simulink model "RobotX_SLAMonly"  (R2014a)
settings: Solver=FixedStepDiscrete  StartTime=0.0  StopTime=inf  FixedStep=.25  RelTol=1e-3
undefined symbols (not defined in the file): Com1, Com2, Com3, Com4, DiscIntNeverNeededParam, standard
libraries: xpcseriallib x11, simulink x3, slrtlib x3, dspmtrx3 x2, speedgoatlib x1, speedgoatlib_IO102 x1
(part 9 of 15)

== system RobotX_SLAMonly/Main FSM/SLAM/Models for prediction/Model40 ==
  X : Inport
  Y : Inport  Port=2
  Psi : Inport  Port=3
  Nav Messages : Inport  Port=4
  Bus Selector : BusSelector  OutputSignals=Velocity.u,Velocity.v,Velocity.r,Port.PtThrust,Port.PtAzimuth,Stbd.StThrust,Stbd.StAzimuth
  Data Store Read : DataStoreRead  DataStoreName=noiseLevel
  Demux : Demux  Outputs=3
  Discrete-Time Integrator1 : DiscreteIntegrator  SampleTime=-1  ICPrevOutput=DiscIntNeverNeededParam  ICPrevScaledInput=DiscIntNeverNeededParam
  Dynamic Model : MATLAB Function  TreatAsAtomicUnit=on
  Mux : Mux  Inputs=3
  Mux1 : Mux  Inputs=3
  Non-Holonomic Constraint : MATLAB Function  TreatAsAtomicUnit=on
  Port Thruster Model : MATLAB Function  TreatAsAtomicUnit=on
  Stbd Thruster Model : MATLAB Function  TreatAsAtomicUnit=on
  Sum : Sum  Inputs=|++|
  enabled : Constant
  move_part : MATLAB Function  TreatAsAtomicUnit=on
  NEyaw : Outport
  wires:
  Sum/1 -> Demux/1  "Forces"
  Bus Selector/2 -> Non-Holonomic Constraint/6(v), Dynamic Model/5(v)  "<v>"
  Bus Selector/1 -> Non-Holonomic Constraint/5(u), Dynamic Model/4(u)  "<u>"
  Psi/1 -> Non-Holonomic Constraint/8(psi), Dynamic Model/6(psi)
  Demux/2 -> Dynamic Model/2(F_sway)
  Demux/3 -> Dynamic Model/3(Torque)
  Demux/1 -> Dynamic Model/1(F_surge)
  Mux/1 -> Sum/2
  Stbd Thruster Model/1(F_surge) -> Mux/1
  Stbd Thruster Model/3(Torque) -> Mux/3
  Stbd Thruster Model/2(F_sway) -> Mux/2
  Mux1/1 -> Sum/1
  Port Thruster Model/2(F_sway) -> Mux1/2
  Port Thruster Model/1(F_surge) -> Mux1/1
  Port Thruster Model/3(Torque) -> Mux1/3
  Dynamic Model/1(surgeAccel) -> Non-Holonomic Constraint/2(surgeAccel)
  Dynamic Model/2(swayAccel) -> Non-Holonomic Constraint/3(swayAccel)
  Dynamic Model/3(yawAccel) -> Non-Holonomic Constraint/4(YawAccel)
  Y/1 -> Non-Holonomic Constraint/10(Y)
  X/1 -> Non-Holonomic Constraint/9(X)
  Bus Selector/3 -> Non-Holonomic Constraint/7(gyrz)  "<r>"
  Non-Holonomic Constraint/1(NEyaw) -> NEyaw/1
  enabled/1 -> Discrete-Time Integrator1/1
  Discrete-Time Integrator1/1 -> Non-Holonomic Constraint/1(time)
  Nav Messages/1 -> Bus Selector/1
  Bus Selector/4 -> move_part/1(PtThrust)  "<PtThrust>"
  Bus Selector/5 -> move_part/2(PtAzimuth)  "<PtAzimuth>"
  Bus Selector/7 -> move_part/4(StAzimuth)  "<StAzimuth>"
  Bus Selector/6 -> move_part/3(StThrust)  "<StThrust>"
  move_part/1(portMP) -> Port Thruster Model/1(portMP)
  move_part/2(portAzimuth) -> Port Thruster Model/2(portAzimuth)
  move_part/3(stbdMP) -> Stbd Thruster Model/1(stbdMP)
  move_part/4(stbdAzimuth) -> Stbd Thruster Model/2(stbdAzimuth)
  Data Store Read/1 -> move_part/5(noiseLevel)

== system RobotX_SLAMonly/Main FSM/SLAM/Models for prediction/Model41 ==
  X : Inport
  Y : Inport  Port=2
  Psi : Inport  Port=3
  Nav Messages : Inport  Port=4
  Bus Selector : BusSelector  OutputSignals=Velocity.u,Velocity.v,Velocity.r,Port.PtThrust,Port.PtAzimuth,Stbd.StThrust,Stbd.StAzimuth
  Data Store Read : DataStoreRead  DataStoreName=noiseLevel
  Demux : Demux  Outputs=3
  Discrete-Time Integrator1 : DiscreteIntegrator  SampleTime=-1  ICPrevOutput=DiscIntNeverNeededParam  ICPrevScaledInput=DiscIntNeverNeededParam
  Dynamic Model : MATLAB Function  TreatAsAtomicUnit=on
  Mux : Mux  Inputs=3
  Mux1 : Mux  Inputs=3
  Non-Holonomic Constraint : MATLAB Function  TreatAsAtomicUnit=on
  Port Thruster Model : MATLAB Function  TreatAsAtomicUnit=on
  Stbd Thruster Model : MATLAB Function  TreatAsAtomicUnit=on
  Sum : Sum  Inputs=|++|
  enabled : Constant
  move_part : MATLAB Function  TreatAsAtomicUnit=on
  NEyaw : Outport
  wires:
  Sum/1 -> Demux/1  "Forces"
  Bus Selector/2 -> Non-Holonomic Constraint/6(v), Dynamic Model/5(v)  "<v>"
  Bus Selector/1 -> Non-Holonomic Constraint/5(u), Dynamic Model/4(u)  "<u>"
  Psi/1 -> Non-Holonomic Constraint/8(psi), Dynamic Model/6(psi)
  Demux/2 -> Dynamic Model/2(F_sway)
  Demux/3 -> Dynamic Model/3(Torque)
  Demux/1 -> Dynamic Model/1(F_surge)
  Mux/1 -> Sum/2
  Stbd Thruster Model/1(F_surge) -> Mux/1
  Stbd Thruster Model/3(Torque) -> Mux/3
  Stbd Thruster Model/2(F_sway) -> Mux/2
  Mux1/1 -> Sum/1
  Port Thruster Model/2(F_sway) -> Mux1/2
  Port Thruster Model/1(F_surge) -> Mux1/1
  Port Thruster Model/3(Torque) -> Mux1/3
  Dynamic Model/1(surgeAccel) -> Non-Holonomic Constraint/2(surgeAccel)
  Dynamic Model/2(swayAccel) -> Non-Holonomic Constraint/3(swayAccel)
  Dynamic Model/3(yawAccel) -> Non-Holonomic Constraint/4(YawAccel)
  Y/1 -> Non-Holonomic Constraint/10(Y)
  X/1 -> Non-Holonomic Constraint/9(X)
  Bus Selector/3 -> Non-Holonomic Constraint/7(gyrz)  "<r>"
  Non-Holonomic Constraint/1(NEyaw) -> NEyaw/1
  enabled/1 -> Discrete-Time Integrator1/1
  Discrete-Time Integrator1/1 -> Non-Holonomic Constraint/1(time)
  Nav Messages/1 -> Bus Selector/1
  Bus Selector/4 -> move_part/1(PtThrust)  "<PtThrust>"
  Bus Selector/5 -> move_part/2(PtAzimuth)  "<PtAzimuth>"
  Bus Selector/7 -> move_part/4(StAzimuth)  "<StAzimuth>"
  Bus Selector/6 -> move_part/3(StThrust)  "<StThrust>"
  move_part/1(portMP) -> Port Thruster Model/1(portMP)
  move_part/2(portAzimuth) -> Port Thruster Model/2(portAzimuth)
  move_part/3(stbdMP) -> Stbd Thruster Model/1(stbdMP)
  move_part/4(stbdAzimuth) -> Stbd Thruster Model/2(stbdAzimuth)
  Data Store Read/1 -> move_part/5(noiseLevel)

== system RobotX_SLAMonly/Main FSM/SLAM/Models for prediction/Model42 ==
  X : Inport
  Y : Inport  Port=2
  Psi : Inport  Port=3
  Nav Messages : Inport  Port=4
  Bus Selector : BusSelector  OutputSignals=Velocity.u,Velocity.v,Velocity.r,Port.PtThrust,Port.PtAzimuth,Stbd.StThrust,Stbd.StAzimuth
  Data Store Read : DataStoreRead  DataStoreName=noiseLevel
  Demux : Demux  Outputs=3
  Discrete-Time Integrator1 : DiscreteIntegrator  SampleTime=-1  ICPrevOutput=DiscIntNeverNeededParam  ICPrevScaledInput=DiscIntNeverNeededParam
  Dynamic Model : MATLAB Function  TreatAsAtomicUnit=on
  Mux : Mux  Inputs=3
  Mux1 : Mux  Inputs=3
  Non-Holonomic Constraint : MATLAB Function  TreatAsAtomicUnit=on
  Port Thruster Model : MATLAB Function  TreatAsAtomicUnit=on
  Stbd Thruster Model : MATLAB Function  TreatAsAtomicUnit=on
  Sum : Sum  Inputs=|++|
  enabled : Constant
  move_part : MATLAB Function  TreatAsAtomicUnit=on
  NEyaw : Outport
  wires:
  Sum/1 -> Demux/1  "Forces"
  Bus Selector/2 -> Non-Holonomic Constraint/6(v), Dynamic Model/5(v)  "<v>"
  Bus Selector/1 -> Non-Holonomic Constraint/5(u), Dynamic Model/4(u)  "<u>"
  Psi/1 -> Non-Holonomic Constraint/8(psi), Dynamic Model/6(psi)
  Demux/2 -> Dynamic Model/2(F_sway)
  Demux/3 -> Dynamic Model/3(Torque)
  Demux/1 -> Dynamic Model/1(F_surge)
  Mux/1 -> Sum/2
  Stbd Thruster Model/1(F_surge) -> Mux/1
  Stbd Thruster Model/3(Torque) -> Mux/3
  Stbd Thruster Model/2(F_sway) -> Mux/2
  Mux1/1 -> Sum/1
  Port Thruster Model/2(F_sway) -> Mux1/2
  Port Thruster Model/1(F_surge) -> Mux1/1
  Port Thruster Model/3(Torque) -> Mux1/3
  Dynamic Model/1(surgeAccel) -> Non-Holonomic Constraint/2(surgeAccel)
  Dynamic Model/2(swayAccel) -> Non-Holonomic Constraint/3(swayAccel)
  Dynamic Model/3(yawAccel) -> Non-Holonomic Constraint/4(YawAccel)
  Y/1 -> Non-Holonomic Constraint/10(Y)
  X/1 -> Non-Holonomic Constraint/9(X)
  Bus Selector/3 -> Non-Holonomic Constraint/7(gyrz)  "<r>"
  Non-Holonomic Constraint/1(NEyaw) -> NEyaw/1
  enabled/1 -> Discrete-Time Integrator1/1
  Discrete-Time Integrator1/1 -> Non-Holonomic Constraint/1(time)
  Nav Messages/1 -> Bus Selector/1
  Bus Selector/4 -> move_part/1(PtThrust)  "<PtThrust>"
  Bus Selector/5 -> move_part/2(PtAzimuth)  "<PtAzimuth>"
  Bus Selector/7 -> move_part/4(StAzimuth)  "<StAzimuth>"
  Bus Selector/6 -> move_part/3(StThrust)  "<StThrust>"
  move_part/1(portMP) -> Port Thruster Model/1(portMP)
  move_part/2(portAzimuth) -> Port Thruster Model/2(portAzimuth)
  move_part/3(stbdMP) -> Stbd Thruster Model/1(stbdMP)
  move_part/4(stbdAzimuth) -> Stbd Thruster Model/2(stbdAzimuth)
  Data Store Read/1 -> move_part/5(noiseLevel)

== system RobotX_SLAMonly/Main FSM/SLAM/Models for prediction/Model43 ==
  X : Inport
  Y : Inport  Port=2
  Psi : Inport  Port=3
  Nav Messages : Inport  Port=4
  Bus Selector : BusSelector  OutputSignals=Velocity.u,Velocity.v,Velocity.r,Port.PtThrust,Port.PtAzimuth,Stbd.StThrust,Stbd.StAzimuth
  Data Store Read : DataStoreRead  DataStoreName=noiseLevel
  Demux : Demux  Outputs=3
  Discrete-Time Integrator1 : DiscreteIntegrator  SampleTime=-1  ICPrevOutput=DiscIntNeverNeededParam  ICPrevScaledInput=DiscIntNeverNeededParam
  Dynamic Model : MATLAB Function  TreatAsAtomicUnit=on
  Mux : Mux  Inputs=3
  Mux1 : Mux  Inputs=3
  Non-Holonomic Constraint : MATLAB Function  TreatAsAtomicUnit=on
  Port Thruster Model : MATLAB Function  TreatAsAtomicUnit=on
  Stbd Thruster Model : MATLAB Function  TreatAsAtomicUnit=on
  Sum : Sum  Inputs=|++|
  enabled : Constant
  move_part : MATLAB Function  TreatAsAtomicUnit=on
  NEyaw : Outport
  wires:
  Sum/1 -> Demux/1  "Forces"
  Bus Selector/2 -> Non-Holonomic Constraint/6(v), Dynamic Model/5(v)  "<v>"
  Bus Selector/1 -> Non-Holonomic Constraint/5(u), Dynamic Model/4(u)  "<u>"
  Psi/1 -> Non-Holonomic Constraint/8(psi), Dynamic Model/6(psi)
  Demux/2 -> Dynamic Model/2(F_sway)
  Demux/3 -> Dynamic Model/3(Torque)
  Demux/1 -> Dynamic Model/1(F_surge)
  Mux/1 -> Sum/2
  Stbd Thruster Model/1(F_surge) -> Mux/1
  Stbd Thruster Model/3(Torque) -> Mux/3
  Stbd Thruster Model/2(F_sway) -> Mux/2
  Mux1/1 -> Sum/1
  Port Thruster Model/2(F_sway) -> Mux1/2
  Port Thruster Model/1(F_surge) -> Mux1/1
  Port Thruster Model/3(Torque) -> Mux1/3
  Dynamic Model/1(surgeAccel) -> Non-Holonomic Constraint/2(surgeAccel)
  Dynamic Model/2(swayAccel) -> Non-Holonomic Constraint/3(swayAccel)
  Dynamic Model/3(yawAccel) -> Non-Holonomic Constraint/4(YawAccel)
  Y/1 -> Non-Holonomic Constraint/10(Y)
  X/1 -> Non-Holonomic Constraint/9(X)
  Bus Selector/3 -> Non-Holonomic Constraint/7(gyrz)  "<r>"
  Non-Holonomic Constraint/1(NEyaw) -> NEyaw/1
  enabled/1 -> Discrete-Time Integrator1/1
  Discrete-Time Integrator1/1 -> Non-Holonomic Constraint/1(time)
  Nav Messages/1 -> Bus Selector/1
  Bus Selector/4 -> move_part/1(PtThrust)  "<PtThrust>"
  Bus Selector/5 -> move_part/2(PtAzimuth)  "<PtAzimuth>"
  Bus Selector/7 -> move_part/4(StAzimuth)  "<StAzimuth>"
  Bus Selector/6 -> move_part/3(StThrust)  "<StThrust>"
  move_part/1(portMP) -> Port Thruster Model/1(portMP)
  move_part/2(portAzimuth) -> Port Thruster Model/2(portAzimuth)
  move_part/3(stbdMP) -> Stbd Thruster Model/1(stbdMP)
  move_part/4(stbdAzimuth) -> Stbd Thruster Model/2(stbdAzimuth)
  Data Store Read/1 -> move_part/5(noiseLevel)

== system RobotX_SLAMonly/Main FSM/SLAM/Models for prediction/Model44 ==
  X : Inport
  Y : Inport  Port=2
  Psi : Inport  Port=3
  Nav Messages : Inport  Port=4
  Bus Selector : BusSelector  OutputSignals=Velocity.u,Velocity.v,Velocity.r,Port.PtThrust,Port.PtAzimuth,Stbd.StThrust,Stbd.StAzimuth
  Data Store Read : DataStoreRead  DataStoreName=noiseLevel
  Demux : Demux  Outputs=3
  Discrete-Time Integrator1 : DiscreteIntegrator  SampleTime=-1  ICPrevOutput=DiscIntNeverNeededParam  ICPrevScaledInput=DiscIntNeverNeededParam
  Dynamic Model : MATLAB Function  TreatAsAtomicUnit=on
  Mux : Mux  Inputs=3
  Mux1 : Mux  Inputs=3
  Non-Holonomic Constraint : MATLAB Function  TreatAsAtomicUnit=on
  Port Thruster Model : MATLAB Function  TreatAsAtomicUnit=on
  Stbd Thruster Model : MATLAB Function  TreatAsAtomicUnit=on
  Sum : Sum  Inputs=|++|
  enabled : Constant
  move_part : MATLAB Function  TreatAsAtomicUnit=on
  NEyaw : Outport
  wires:
  Sum/1 -> Demux/1  "Forces"
  Bus Selector/2 -> Non-Holonomic Constraint/6(v), Dynamic Model/5(v)  "<v>"
  Bus Selector/1 -> Non-Holonomic Constraint/5(u), Dynamic Model/4(u)  "<u>"
  Psi/1 -> Non-Holonomic Constraint/8(psi), Dynamic Model/6(psi)
  Demux/2 -> Dynamic Model/2(F_sway)
  Demux/3 -> Dynamic Model/3(Torque)
  Demux/1 -> Dynamic Model/1(F_surge)
  Mux/1 -> Sum/2
  Stbd Thruster Model/1(F_surge) -> Mux/1
  Stbd Thruster Model/3(Torque) -> Mux/3
  Stbd Thruster Model/2(F_sway) -> Mux/2
  Mux1/1 -> Sum/1
  Port Thruster Model/2(F_sway) -> Mux1/2
  Port Thruster Model/1(F_surge) -> Mux1/1
  Port Thruster Model/3(Torque) -> Mux1/3
  Dynamic Model/1(surgeAccel) -> Non-Holonomic Constraint/2(surgeAccel)
  Dynamic Model/2(swayAccel) -> Non-Holonomic Constraint/3(swayAccel)
  Dynamic Model/3(yawAccel) -> Non-Holonomic Constraint/4(YawAccel)
  Y/1 -> Non-Holonomic Constraint/10(Y)
  X/1 -> Non-Holonomic Constraint/9(X)
  Bus Selector/3 -> Non-Holonomic Constraint/7(gyrz)  "<r>"
  Non-Holonomic Constraint/1(NEyaw) -> NEyaw/1
  enabled/1 -> Discrete-Time Integrator1/1
  Discrete-Time Integrator1/1 -> Non-Holonomic Constraint/1(time)
  Nav Messages/1 -> Bus Selector/1
  Bus Selector/4 -> move_part/1(PtThrust)  "<PtThrust>"
  Bus Selector/5 -> move_part/2(PtAzimuth)  "<PtAzimuth>"
  Bus Selector/7 -> move_part/4(StAzimuth)  "<StAzimuth>"
  Bus Selector/6 -> move_part/3(StThrust)  "<StThrust>"
  move_part/1(portMP) -> Port Thruster Model/1(portMP)
  move_part/2(portAzimuth) -> Port Thruster Model/2(portAzimuth)
  move_part/3(stbdMP) -> Stbd Thruster Model/1(stbdMP)
  move_part/4(stbdAzimuth) -> Stbd Thruster Model/2(stbdAzimuth)
  Data Store Read/1 -> move_part/5(noiseLevel)

== system RobotX_SLAMonly/Main FSM/SLAM/Models for prediction/Model45 ==
  X : Inport
  Y : Inport  Port=2
  Psi : Inport  Port=3
  Nav Messages : Inport  Port=4
  Bus Selector : BusSelector  OutputSignals=Velocity.u,Velocity.v,Velocity.r,Port.PtThrust,Port.PtAzimuth,Stbd.StThrust,Stbd.StAzimuth
  Data Store Read : DataStoreRead  DataStoreName=noiseLevel
  Demux : Demux  Outputs=3
  Discrete-Time Integrator1 : DiscreteIntegrator  SampleTime=-1  ICPrevOutput=DiscIntNeverNeededParam  ICPrevScaledInput=DiscIntNeverNeededParam
  Dynamic Model : MATLAB Function  TreatAsAtomicUnit=on
  Mux : Mux  Inputs=3
  Mux1 : Mux  Inputs=3
  Non-Holonomic Constraint : MATLAB Function  TreatAsAtomicUnit=on
  Port Thruster Model : MATLAB Function  TreatAsAtomicUnit=on
  Stbd Thruster Model : MATLAB Function  TreatAsAtomicUnit=on
  Sum : Sum  Inputs=|++|
  enabled : Constant
  move_part : MATLAB Function  TreatAsAtomicUnit=on
  NEyaw : Outport
  wires:
  Sum/1 -> Demux/1  "Forces"
  Bus Selector/2 -> Non-Holonomic Constraint/6(v), Dynamic Model/5(v)  "<v>"
  Bus Selector/1 -> Non-Holonomic Constraint/5(u), Dynamic Model/4(u)  "<u>"
  Psi/1 -> Non-Holonomic Constraint/8(psi), Dynamic Model/6(psi)
  Demux/2 -> Dynamic Model/2(F_sway)
  Demux/3 -> Dynamic Model/3(Torque)
  Demux/1 -> Dynamic Model/1(F_surge)
  Mux/1 -> Sum/2
  Stbd Thruster Model/1(F_surge) -> Mux/1
  Stbd Thruster Model/3(Torque) -> Mux/3
  Stbd Thruster Model/2(F_sway) -> Mux/2
  Mux1/1 -> Sum/1
  Port Thruster Model/2(F_sway) -> Mux1/2
  Port Thruster Model/1(F_surge) -> Mux1/1
  Port Thruster Model/3(Torque) -> Mux1/3
  Dynamic Model/1(surgeAccel) -> Non-Holonomic Constraint/2(surgeAccel)
  Dynamic Model/2(swayAccel) -> Non-Holonomic Constraint/3(swayAccel)
  Dynamic Model/3(yawAccel) -> Non-Holonomic Constraint/4(YawAccel)
  Y/1 -> Non-Holonomic Constraint/10(Y)
  X/1 -> Non-Holonomic Constraint/9(X)
  Bus Selector/3 -> Non-Holonomic Constraint/7(gyrz)  "<r>"
  Non-Holonomic Constraint/1(NEyaw) -> NEyaw/1
  enabled/1 -> Discrete-Time Integrator1/1
  Discrete-Time Integrator1/1 -> Non-Holonomic Constraint/1(time)
  Nav Messages/1 -> Bus Selector/1
  Bus Selector/4 -> move_part/1(PtThrust)  "<PtThrust>"
  Bus Selector/5 -> move_part/2(PtAzimuth)  "<PtAzimuth>"
  Bus Selector/7 -> move_part/4(StAzimuth)  "<StAzimuth>"
  Bus Selector/6 -> move_part/3(StThrust)  "<StThrust>"
  move_part/1(portMP) -> Port Thruster Model/1(portMP)
  move_part/2(portAzimuth) -> Port Thruster Model/2(portAzimuth)
  move_part/3(stbdMP) -> Stbd Thruster Model/1(stbdMP)
  move_part/4(stbdAzimuth) -> Stbd Thruster Model/2(stbdAzimuth)
  Data Store Read/1 -> move_part/5(noiseLevel)

== matlab function RobotX_SLAMonly/Main FSM/Path/A Star (Held Length) ==
  data: relPose input; Path output; obGrid input; targetPt input
function Path  = AStarHeldLengthDebug( relPose, obGrid, targetPt )
%Written By Anderson Lebbad on August 27, 2014
%Last Edited on:

%This funtion executes an A* method for path planning given the current
%position of the vessel, the target position for the vessel to reach, and
%a map of obstacles to avoid. The A* method is well documented here:
% www.policyalmanac.org/games/aStarTutorial.htm

%% Define list sizes
[m,n] = size(obGrid);
gridPts = m*n;

%Initialize a path output variable
Path = nan(gridPts,2);
%Initialize variable to track if a solution has been found
solution_found = 0;

%Track the XY coordinates of each point to be evaluated
open_list_XY = nan(gridPts,2);
%Track the calculated F, G, and H weights (where G is the movement cost to
%get to the point, H is the Hypothetical cost to reach the target from that
%point before the full path is evaluated, and F is the sum of both G and H
%costs) for the points being evaluated
open_list_FGH = nan(gridPts,3);
%Track the coordinates of the parent for each of the points being evaluated
open_list_parent = nan(gridPts,2);

%Track the XY coordinates of each point that has been fully evaluated
closed_list_XY = nan(gridPts,2);
%Track the parent coordinate of each point that has been fully evaluated
closed_list_parent = nan(gridPts,2);
emptyClosed = find(isnan(closed_list_XY(:,1)));

%Relative indices to neighboring points of the square, to be used for
%evaluating potential candidates for the open list
neighbors_XY = [-1,-1;-1,0;-1,1;0,1;1,1;1,0;1,-1;0,-1];
neighbors_G = [14;10;14;10;14;10;14;10];

%Make the current pose (in the relative coordinates of the field) the first
%point in the open list
open_list_XY(1,:) = relPose;
current_XY = relPose;
%Set movement cost of this point to zero
open_list_FGH(1,2) = 0;
%Calculate hypothetical cost
open_list_FGH(1,3) = 10*(abs(targetPt(1)-relPose(1))+abs(targetPt(2)-relPose(2)));
%Sum is full cost
open_list_FGH(1,1) = open_list_FGH(1,2) + open_list_FGH(1,3);

%Create a list of invalid pts
%obstacles are invalid
[row, col] = find(obGrid == -1);
%outside the edges are invalid
left = [0:m+1;zeros(1,m+2)]';
right = [0:m+1;(n+1)*ones(1,m+2)]';
bottom = [zeros(1,n);1:n]';
top = [(m+1)*ones(1,n);1:n]';
invalid_pts = [row,col;left;right;bottom;top];
invalid_pts = sortrows(invalid_pts);
%Loop while there are points on the open list
while sum(~isnan(open_list_XY(:,1))) >= 1
    %% Current Square
    
    %Find the lowest F cost square on the open list, checking newer entries
    %over older. This is done by flipping the list up/down to get newer
    %entries to evaluate first. This is marked as the current square
    [~,idxI] = min(flipud(open_list_FGH(:,1)));
    CurrentSquare = gridPts - idxI(1) + 1;
    current_XY = open_list_XY(CurrentSquare,:);
    current_G = open_list_FGH(CurrentSquare,2);
    
    %Find the first empty element in the closed list, and replace the place
    %holder with the information for the current square
    emptyClosed = find(isnan(closed_list_XY(:,1)));
    closed_list_XY(emptyClosed(1),:) = current_XY;
    closed_list_parent(emptyClosed(1),:) = open_list_parent(CurrentSquare,:);
    %Remove the current square from the open list now that it is on the
    %closed list
    open_list_XY(CurrentSquare,:) = NaN;
    open_list_FGH(CurrentSquare,:) = NaN;
    open_list_parent(CurrentSquare,:) = NaN;
    
    %If the current point that just got added to the closed list is the
    %target point, exit the loop because a complete path can be traced
    if (current_XY(1) == targetPt(1)) && (current_XY(2) == targetPt(2))
        solution_found = 1;
        break
    end
    
    %% Check adjacent squares
    
    %Create a list of points around the current point and check their G
    %value
    rel_list_XY = [neighbors_XY(:,1)+current_XY(1) neighbors_XY(:,2)+current_XY(2)];
    rel_list_G = neighbors_G + current_G;
    rel_list_H = 10*(abs(targetPt(1)-rel_list_XY(:,1))+abs(targetPt(2)-rel_list_XY(:,2)));
    rel_list_F = rel_list_G + rel_list_H;
    
    %% Check walkable / on closed list
    
    %Order closed list for finding relative list points on it
    closed_list_XY_sorted = sortrows(closed_list_XY);
    %Mark members of relative list if on closed list
    on_closed = ismember(rel_list_XY,closed_list_XY_sorted,'rows');
    rel_list_XY(on_closed,:) = NaN;
    rel_list_F(on_closed) = NaN;
    rel_list_G(on_closed) = NaN;
    rel_list_H(on_closed) = NaN;
    %Check to see if members of relative list are either obstacles or out
    %of bounds
    invalid = ismember(rel_list_XY,invalid_pts,'rows');
    rel_list_XY(invalid,:) = NaN;
    rel_list_F(invalid) = NaN;
    rel_list_G(invalid) = NaN;
    rel_list_H(invalid) = NaN;
    valid = ~isnan(rel_list_XY(:,1));
    validIdx = find(valid);
    
    %% Calculate F and H, and add penalty weights to G scores
    
    if ~isempty(rel_list_XY)
        rel_list_G(valid) = rel_list_G(valid) + 20.*obGrid(rel_list_XY(valid,1)+m*(rel_list_XY(valid,2)-1));
        rel_list_F(valid) = rel_list_G(valid) + rel_list_H(valid);
        
        %% Check if on open list, if not add to it
        
        %Order open list for finding relative list points on it
        [open_list_XY_sorted, idx] = sortrows(open_list_XY);
        %Check to see if relative list points are on open list
        [rel_on_open, open_on_rel_list] = ismember(rel_list_XY(valid,:),open_list_XY_sorted,'rows');
        rel_not_on_open = validIdx(~rel_on_open);
        rel_on_open = validIdx(rel_on_open);
        %Only care about indices that are actually found, remove the ones that
        %aren't
        open_on_rel = idx(open_on_rel_list(open_on_rel_list ~= 0));
        %Whichever points that are not on the open list are
        %added to the open list (in the first available empty slots)
        num_not_on_open = length(rel_not_on_open);
        num_on_open = length(rel_on_open);
        emptyOpen = find(isnan(open_list_XY(:,1)));
        if num_not_on_open >= 1
            open_list_XY(emptyOpen(1:num_not_on_open),:) = rel_list_XY(rel_not_on_open,:);
            open_list_FGH(emptyOpen(1:num_not_on_open),:) = ...
                [rel_list_F(rel_not_on_open) rel_list_G(rel_not_on_open) rel_list_H(rel_not_on_open)];
            open_list_parent(emptyOpen(1:num_not_on_open),1) = current_XY(1);
            open_list_parent(emptyOpen(1:num_not_on_open),2) = current_XY(2);
            %Remove members of the relative list that were just put on the open
            %list (only care about the F and G, the XY and H are not updated past
            %this point)
            rel_list_F(~rel_on_open) = NaN;
            rel_list_G(~rel_on_open) = NaN;
        end
        
        %% Check G cost of rest to see if it should be updated
        
        if num_on_open >= 1
            %Find the G values of the points that are on the open list and compare
            %them to the G values for the same points on the relative list. Track
            %which G values are lower on the relative list
            lower_G_list = rel_list_G(rel_on_open) < open_list_FGH(open_on_rel,2);
            rel_idx = find(rel_on_open);
            lower_G = rel_idx(lower_G_list);
            %Replace the G and F values with the new lower ones, and update parent
            open_list_FGH(open_on_rel(lower_G_list),1:2) = [rel_list_F(lower_G) rel_list_G(lower_G)];
            open_list_parent(open_on_rel(lower_G_list),1) = current_XY(1);
            open_list_parent(open_on_rel(lower_G_list),2) = current_XY(2);
        end
        
    end
    
    %% Organize list for searching
    
    %Negates the F and H cost for to be able to descending rowsort, then negates
    %back to original values
    open_list_FGH = -open_list_FGH;
    [open_list_FGH,idx] = sortrows(open_list_FGH,[1 3]); %Sort focusing on F first, then H
    open_list_FGH = -open_list_FGH;
    open_list_XY = open_list_XY(idx,:);
    open_list_parent = open_list_parent(idx,:);
    
end

%% If solution is found, generate path

%Generate path by recursively checking parent values
if solution_found
    %Create a list of the path points, for organizational purposes for
    %outputting later
    PathList = Path;
    %Set first element as current position (the goal point)
    PathList(1,:) = current_XY;
    %Track current square's location on closed list
    CurrentSquareClosed = emptyClosed(1);
    %Create an incrementing variable for path elements
    next_index = 2;
    %Loop until there is no parent square (start square)
    while ~isnan(closed_list_parent(CurrentSquareClosed))
        %Next path element is the current element's parent
        PathList(next_index,:) = closed_list_parent(CurrentSquareClosed,:);
        %Order closed list for finding parents on it
        [closed_list_XY_sorted, idx] = sortrows(closed_list_XY);
        %Find the next element and make it the current element
        [~,locs] = ismember(closed_list_parent(CurrentSquareClosed,:),closed_list_XY_sorted,'rows');
        CurrentSquareClosed = idx(locs(1));
        %Increment the next index
        next_index = next_index + 1;
    end
    %Get the length of the path
    PathLength = next_index-1;
    %Path list is from finish to start, so flip and output
    Path(1:PathLength,:) = PathList(PathLength:-1:1,:);
end

end

== matlab function RobotX_SLAMonly/Main FSM/SLAM/Models for prediction/Model10/Port Thruster Model ==
  data: portMP input; F_surge output; portAzimuth input; F_sway output; Torque output
function [F_surge,F_sway,Torque]  = PortThruster(portMP,portAzimuth)
%Approximation for Starboard Force and Moment with the input motor power
%and azimuth angle of thruster

%Longitudinal distance from center of mass
longDist =1.007;           %m

%Axial distance from center of mass
axialDist=1.485;            %m

%% Piece-wise thrust calculation

if portMP <= -51.0119
    F = .9140*portMP + 40;
elseif portMP >= 26.8367
    F = 1.658*portMP - 41.01;
else
    F = .12987*portMP;
end

%% Force components
F_surge=F*cos(portAzimuth*pi/180);       %N
F_sway=F*sin(portAzimuth*pi/180);       %N

%% Torque calculation

Torque = F_surge*longDist - F_sway*axialDist;   %N.m

end

== matlab function RobotX_SLAMonly/Main FSM/SLAM/Models for prediction/Model10/Stbd Thruster Model ==
  data: stbdMP input; F_surge output; stbdAzimuth input; F_sway output; Torque output
function [F_surge,F_sway,Torque]  = StarBoardThruster(stbdMP,stbdAzimuth)
%Approximation for Starboard Force and Moment with the input motor power
%and azimuth angle of thruster

%Longitudinal distance from center of mass
longDist =1.007;           %m

%Axial distance from center of mass
axialDist=1.485;            %m

%% Piece-wise thrust calculation

if stbdMP <= -51.0119
    F = .9140*stbdMP + 40;
elseif stbdMP >= 26.8367
    F = 1.658*stbdMP - 41.01;
else
    F = .12987*stbdMP;
end

%% Force components
F_surge=F*cos(stbdAzimuth*pi/180);       %N
F_sway=F*sin(stbdAzimuth*pi/180);       %N

%% Torque calculation

Torque = -F_surge*longDist - F_sway*axialDist;   %N.m

end

== matlab function RobotX_SLAMonly/Main FSM/SLAM/Models for prediction/Model6/Dynamic Model ==
  data: F_surge input; F_sway input; Torque input; u input; surgeAccel output; v input; psi input; swayAccel output; yawAccel output
function [surgeAccel, swayAccel, yawAccel] = ...
    WAM_V_3DOF(F_surge, F_sway, Torque, u, v, psi)
%Written by Anderson Lebbad on August 12, 2014
%Last Edited:

%This function was heavily based off of Ariel Qu's Vel3DOF_IvanV1. It was
%rewritten for real-time use.

%This function will produce the transient output surge velocity of a
%linearized model of the USV. It is assumed that the vehicle is equivalent
%to two cylinders in the water.

%%%%%DEFINED VARIABLE%%%%%%
%
%   Xext = Thrust from motors
%   Next = Moment from motor
%   m = Mass of vehicle
%   Xudot = Added mass in surge direction
%   Yvdot = Added mass in sway direction
%   Nrdot = Added mass from yaw
%   xg = offset from center of gravity
%   rho = density of seawater
%   S = wetted surface area
%   R = Reynolds number
%   Cd = Coefficient of drag
%   Cdc = Coefficient of drag for sway
%   nu = Kinematic viscosity
%   L = Length overall
%   T = draft
%   B = beam
%   SA = Surface area of cylinder experiencing sway
%   Iz = moment of inertia about Z axis
%
%%%%%%

% Force/Mometns from thrusters & control surfaces...

tau = [F_surge; F_sway; Torque];

% Calculate yaw rate
persistent lastHeading
if isempty(lastHeading)
    lastHeading = psi;
end
%Sample time
ts = .1;

r = (psi - lastHeading)/ts;

% Velocity & Angular velocity vectors
vel = [u; v; 0];
omega = [0; 0; r];

%define variables
m = 145.7;         % Total mass [kg] - reduced from 102
rho = 1025.9;   % density of seawater [kg/m^3]
L = 3.91*0.85;  % Length on the waterline [m]
B = 0.426;       % Demihull beam [m]
T = B*0.2;        % Draft of the demihull [m]
p_bar = 1.0; % sidehull separation - from centerplane vessel to centerplane demihull
Iz = 262.181;    % Mass moment of inertia about z-axis [kg*m^2]
xg = 0;         % Body-Fixed coordinate system taken to be center of gravity
yg = 0;         % Symmetrical Vessel
Cd = 1.1;       % Drag coefficient for a lateral cylinder
LCG = 1.485;        % Need to know where LCG wrt stern

% Vector location of port and starboard hulls
r_port = [-LCG; -p_bar; 0];   
r_stbd = [-LCG; p_bar; 0];

% Port and starboard hull velocities
vel_port = vel + cross(omega,r_port);
vel_stbd = vel + cross(omega,r_stbd);

u_port = vel_port(1);
u_stbd = vel_stbd(1);

% Port and starboard state vectors
state_port = vel_port + omega;
state_stbd = vel_stbd + omega;

%% Added Mass
% Estimated for each hull, then multiplied by 2 to account for both hulls
Xudot = -0.05*m;

%Using strip theory to estimate added mass coefficients
Nrdot = -(4.75/2*pi*rho*p_bar*T^4 + pi*rho*T^2*((L - LCG)^3 + LCG^3)/3);
Nvdot = - pi*rho*T^2*((L - LCG)^2 - LCG^2)/2;

Yrdot = Nvdot;
Yvdot = -rho*pi*T^2*L;

% Multiply by 2:
Xudot = 2*Xudot;
Nrdot = 2*Nrdot;
Nvdot = 2*Nvdot;
Yrdot = 2*Yrdot;
Yvdot = 2*Yvdot;

%Calculate Coefficient of Drag for Sway from 1950 SNAME approximation
Cdc= 1.1 + 0.0045*L/T - 0.1*B/T + 0.016*(B/T)^2;
SA = 2*pi/4*T*L; %projected area of pontoon for two pontoons

%% Linear Drag Terms
%Total Speed
U = sqrt(u^2+v^2);

Xu = 0;
Yv = -0.5*rho*abs(v)*2*Cdc*SA; %20 was the last working number %from SNAME 1950, x2 for two cylinders
%Nr = -0.5*pi*rho*U*T^2*L^2;
Nr = -pi*rho*U*T^2*L^2*.065;
Nv = -pi*rho*U*T^2*L*.01;
Yr = pi*rho*U*T^2*L*0.2;  %from Newman approximation in Lewandowski

%% Nonlinear Drag Terms

% Drag and Moment due to drag on entire vessel - includes nonlinear and
% linear drag terms
D_port = 0.5*(0.44*u_port^3 - 0.01*u_port^2 + 19*u_port);     % Can assume that this equation also takes into account Xu - so set Xu=0
D_stbd = 0.5*(0.44*u_stbd^3 - 0.01*u_stbd^2 + 19*u_stbd);     % Can assume that this equation also takes into account Xu - so set Xu=0

tau_drag = [-(D_port + D_stbd); 0; (D_stbd - D_port)*p_bar];

Xuu = 0;

%% Maneuvering Coefficient Matrices
% Added Mass Matrix
M = [(m - Xudot)      0              0;...
    0               (m - Yvdot)     (m*xg - Yrdot);...
    0               (m*xg - Nvdot)  (Iz - Nrdot)];

%Centripetal and Added Mass Centripetal force matrices
% C_RB = [
%     0                  0                0
%     0                  0                0
%     0                  0                0
%     ];

% C_RB = [
%     0                  0                -m*(xg*r + v)
%     0                  0                -m*(yg*r - u)
%     m*(xg*r + v)       m*(yg*r - u)     0
%     ];

% C_A = -[ %negative originally
%     0                               0           0
%     0                               0           0
%     0                               0           0
%     ];

% Negating centripetal acceleration for test
C_RB = 0;
C_A = 0;

D = -[Xu  0   0;...
      0   Yv  Yr;...
      0   Nv  Nr];

% Nonlinear Drag Coefficients
D_N = -[Xuu*u   0                       0;...
        0       0                       0;...
        0       0                       0];
    
%% Calculate the port and starboard force vectors
tau_port = -(C_RB + C_A + D + D_N)*state_port;
tau_stbd = -(C_RB + C_A + D + D_N)*state_stbd;


%% Sum the force vectors
tau_tot = tau + tau_drag + tau_port + tau_stbd...
    + cross(r_port,[tau_port(1);tau_port(2);0]) + ...
    cross(r_stbd,[tau_stbd(1);tau_stbd(2);0]);

% Calculate the time derivative of the state vector

accel = M\tau_tot;

%% Separate output

surgeAccel = accel(1);
swayAccel = accel(2);
yawAccel = accel(3);

end

== matlab function RobotX_SLAMonly/Main FSM/SLAM/Models for prediction/Model8/Port Thruster Model ==
  data: portMP input; F_surge output; portAzimuth input; F_sway output; Torque output
function [F_surge,F_sway,Torque]  = PortThruster(portMP,portAzimuth)
%Approximation for Starboard Force and Moment with the input motor power
%and azimuth angle of thruster

%Longitudinal distance from center of mass
longDist =1.007;           %m

%Axial distance from center of mass
axialDist=1.485;            %m

%% Piece-wise thrust calculation

if portMP <= -51.0119
    F = .9140*portMP + 40;
elseif portMP >= 26.8367
    F = 1.658*portMP - 41.01;
else
    F = .12987*portMP;
end

%% Force components
F_surge=F*cos(portAzimuth*pi/180);       %N
F_sway=F*sin(portAzimuth*pi/180);       %N

%% Torque calculation

Torque = F_surge*longDist - F_sway*axialDist;   %N.m

end

== matlab function RobotX_SLAMonly/Main FSM/SLAM/Models for prediction/Model8/Stbd Thruster Model ==
  data: stbdMP input; F_surge output; stbdAzimuth input; F_sway output; Torque output
function [F_surge,F_sway,Torque]  = StarBoardThruster(stbdMP,stbdAzimuth)
%Approximation for Starboard Force and Moment with the input motor power
%and azimuth angle of thruster

%Longitudinal distance from center of mass
longDist =1.007;           %m

%Axial distance from center of mass
axialDist=1.485;            %m

%% Piece-wise thrust calculation

if stbdMP <= -51.0119
    F = .9140*stbdMP + 40;
elseif stbdMP >= 26.8367
    F = 1.658*stbdMP - 41.01;
else
    F = .12987*stbdMP;
end

%% Force components
F_surge=F*cos(stbdAzimuth*pi/180);       %N
F_sway=F*sin(stbdAzimuth*pi/180);       %N

%% Torque calculation

Torque = -F_surge*longDist - F_sway*axialDist;   %N.m

end

== matlab function RobotX_SLAMonly/Main FSM/SLAM/Models for prediction/Model9/Non-Holonomic Constraint ==
  data: time input; surgeAccel input; NEyaw output; swayAccel input; YawAccel input; u input; v input; gyrz input; psi input; X input; Y input
function NEyaw  = nonHolonomicNE(time,surgeAccel,swayAccel,YawAccel,u,v,gyrz,psi,X,Y)
%Written by Anderson Lebbad on August 12, 2014
%Last Edited:

%This function estimates the velocities for a new pose based off the 
%velocities and heading calculated from the dynamic model, and the current 
%pose. Uses a non-holonomic constraint for estimation.

%% Find time elapsed for integration

ts = .1;
persistent uPrev vPrev gyrzPrev psiPrev xPrev yPrev

%Initialize
if isempty(uPrev)
    uPrev = [u time];
    vPrev = [v time];
    gyrzPrev = [gyrz time];
    psiPrev = [psi time];
    xPrev = [X time];
    yPrev = [Y time];
end
    
%Update if change
if uPrev(1) ~= u
    uPrev = [u time];
end
if vPrev(1) ~= v
    vPrev = [v time];
end
if gyrzPrev(1) ~= gyrz
    gyrzPrev = [gyrz time];
end
if psiPrev(1) ~= psi
    psiPrev = [psi time];
end
if xPrev(1) ~= X
    xPrev = [X time];
end
if yPrev(1) ~= Y
    yPrev = [Y time];
end

%evaluate elapsed
uTime = ts + time - uPrev(2);
vTime = ts + time - vPrev(2);
gyrzTime = ts + time - gyrzPrev(2);
psiTime = ts + time - psiPrev(2);
xTime = ts + time - xPrev(2);
yTime = ts + time - yPrev(2);

%% Integrate inputs
surgeVel = u + surgeAccel*uTime/2;
swayVel = v + swayAccel*vTime/2;
yawVel = gyrz + YawAccel*gyrzTime/2;
yaw = psi + yawVel*psiTime/2;


%% Apply Non-holonomic constraint for NE velocities
Xd = surgeVel*cos(yaw*pi/180) - swayVel*sin(yaw*pi/180);
Yd = surgeVel*sin(yaw*pi/180) + swayVel*cos(yaw*pi/180);

%% Integrate to output NE coordinates
N = X + Xd*xTime/2;
E = Y + Yd*yTime/2;

NEyaw = [N;E;yaw];

end

== matlab function RobotX_SLAMonly/Main FSM/SLAM/Models for prediction/Model9/move_part ==
  data: PtThrust input; portMP output; PtAzimuth input; StThrust input; StAzimuth input; noiseLevel input; portAzimuth output; stbdMP output; stbdAzimuth output
function [portMP,portAzimuth,stbdMP,stbdAzimuth] = addNoise(PtThrust,...
    PtAzimuth,StThrust,StAzimuth,noiseLevel)
%Written By Anderson Lebbad on September 16, 2014
%Last Edited By:

%This function adds gaussian noise to the inputs for a particular particles
%model

portMP = normrnd(PtThrust, noiseLevel);
portAzimuth = normrnd(PtAzimuth, noiseLevel);
stbdMP = normrnd(StThrust, noiseLevel);
stbdAzimuth = normrnd(StAzimuth, noiseLevel);

end

== matlab function RobotX_SLAMonly/Main FSM/SLAM/Models for prediction/Model11/Non-Holonomic Constraint ==
  data: time input; surgeAccel input; NEyaw output; swayAccel input; YawAccel input; u input; v input; gyrz input; psi input; X input; Y input
function NEyaw  = nonHolonomicNE(time,surgeAccel,swayAccel,YawAccel,u,v,gyrz,psi,X,Y)
%Written by Anderson Lebbad on August 12, 2014
%Last Edited:

%This function estimates the velocities for a new pose based off the 
%velocities and heading calculated from the dynamic model, and the current 
%pose. Uses a non-holonomic constraint for estimation.

%% Find time elapsed for integration

ts = .1;
persistent uPrev vPrev gyrzPrev psiPrev xPrev yPrev

%Initialize
if isempty(uPrev)
    uPrev = [u time];
    vPrev = [v time];
    gyrzPrev = [gyrz time];
    psiPrev = [psi time];
    xPrev = [X time];
    yPrev = [Y time];
end
    
%Update if change
if uPrev(1) ~= u
    uPrev = [u time];
end
if vPrev(1) ~= v
    vPrev = [v time];
end
if gyrzPrev(1) ~= gyrz
    gyrzPrev = [gyrz time];
end
if psiPrev(1) ~= psi
    psiPrev = [psi time];
end
if xPrev(1) ~= X
    xPrev = [X time];
end
if yPrev(1) ~= Y
    yPrev = [Y time];
end

%evaluate elapsed
uTime = ts + time - uPrev(2);
vTime = ts + time - vPrev(2);
gyrzTime = ts + time - gyrzPrev(2);
psiTime = ts + time - psiPrev(2);
xTime = ts + time - xPrev(2);
yTime = ts + time - yPrev(2);

%% Integrate inputs
surgeVel = u + surgeAccel*uTime/2;
swayVel = v + swayAccel*vTime/2;
yawVel = gyrz + YawAccel*gyrzTime/2;
yaw = psi + yawVel*psiTime/2;


%% Apply Non-holonomic constraint for NE velocities
Xd = surgeVel*cos(yaw*pi/180) - swayVel*sin(yaw*pi/180);
Yd = surgeVel*sin(yaw*pi/180) + swayVel*cos(yaw*pi/180);

%% Integrate to output NE coordinates
N = X + Xd*xTime/2;
E = Y + Yd*yTime/2;

NEyaw = [N;E;yaw];

end

== matlab function RobotX_SLAMonly/Main FSM/SLAM/Models for prediction/Model11/move_part ==
  data: PtThrust input; portMP output; PtAzimuth input; StThrust input; StAzimuth input; noiseLevel input; portAzimuth output; stbdMP output; stbdAzimuth output
function [portMP,portAzimuth,stbdMP,stbdAzimuth] = addNoise(PtThrust,...
    PtAzimuth,StThrust,StAzimuth,noiseLevel)
%Written By Anderson Lebbad on September 16, 2014
%Last Edited By:

%This function adds gaussian noise to the inputs for a particular particles
%model

portMP = normrnd(PtThrust, noiseLevel);
portAzimuth = normrnd(PtAzimuth, noiseLevel);
stbdMP = normrnd(StThrust, noiseLevel);
stbdAzimuth = normrnd(StAzimuth, noiseLevel);

end

== matlab function RobotX_SLAMonly/Main FSM/SLAM/Models for prediction/Model12/Dynamic Model ==
  data: F_surge input; F_sway input; Torque input; u input; surgeAccel output; v input; psi input; swayAccel output; yawAccel output
function [surgeAccel, swayAccel, yawAccel] = ...
    WAM_V_3DOF(F_surge, F_sway, Torque, u, v, psi)
%Written by Anderson Lebbad on August 12, 2014
%Last Edited:

%This function was heavily based off of Ariel Qu's Vel3DOF_IvanV1. It was
%rewritten for real-time use.

%This function will produce the transient output surge velocity of a
%linearized model of the USV. It is assumed that the vehicle is equivalent
%to two cylinders in the water.

%%%%%DEFINED VARIABLE%%%%%%
%
%   Xext = Thrust from motors
%   Next = Moment from motor
%   m = Mass of vehicle
%   Xudot = Added mass in surge direction
%   Yvdot = Added mass in sway direction
%   Nrdot = Added mass from yaw
%   xg = offset from center of gravity
%   rho = density of seawater
%   S = wetted surface area
%   R = Reynolds number
%   Cd = Coefficient of drag
%   Cdc = Coefficient of drag for sway
%   nu = Kinematic viscosity
%   L = Length overall
%   T = draft
%   B = beam
%   SA = Surface area of cylinder experiencing sway
%   Iz = moment of inertia about Z axis
%
%%%%%%

% Force/Mometns from thrusters & control surfaces...

tau = [F_surge; F_sway; Torque];

% Calculate yaw rate
persistent lastHeading
if isempty(lastHeading)
    lastHeading = psi;
end
%Sample time
ts = .1;

r = (psi - lastHeading)/ts;

% Velocity & Angular velocity vectors
vel = [u; v; 0];
omega = [0; 0; r];

%define variables
m = 145.7;         % Total mass [kg] - reduced from 102
rho = 1025.9;   % density of seawater [kg/m^3]
L = 3.91*0.85;  % Length on the waterline [m]
B = 0.426;       % Demihull beam [m]
T = B*0.2;        % Draft of the demihull [m]
p_bar = 1.0; % sidehull separation - from centerplane vessel to centerplane demihull
Iz = 262.181;    % Mass moment of inertia about z-axis [kg*m^2]
xg = 0;         % Body-Fixed coordinate system taken to be center of gravity
yg = 0;         % Symmetrical Vessel
Cd = 1.1;       % Drag coefficient for a lateral cylinder
LCG = 1.485;        % Need to know where LCG wrt stern

% Vector location of port and starboard hulls
r_port = [-LCG; -p_bar; 0];   
r_stbd = [-LCG; p_bar; 0];

% Port and starboard hull velocities
vel_port = vel + cross(omega,r_port);
vel_stbd = vel + cross(omega,r_stbd);

u_port = vel_port(1);
u_stbd = vel_stbd(1);

% Port and starboard state vectors
state_port = vel_port + omega;
state_stbd = vel_stbd + omega;

%% Added Mass
% Estimated for each hull, then multiplied by 2 to account for both hulls
Xudot = -0.05*m;

%Using strip theory to estimate added mass coefficients
Nrdot = -(4.75/2*pi*rho*p_bar*T^4 + pi*rho*T^2*((L - LCG)^3 + LCG^3)/3);
Nvdot = - pi*rho*T^2*((L - LCG)^2 - LCG^2)/2;

Yrdot = Nvdot;
Yvdot = -rho*pi*T^2*L;

% Multiply by 2:
Xudot = 2*Xudot;
Nrdot = 2*Nrdot;
Nvdot = 2*Nvdot;
Yrdot = 2*Yrdot;
Yvdot = 2*Yvdot;

%Calculate Coefficient of Drag for Sway from 1950 SNAME approximation
Cdc= 1.1 + 0.0045*L/T - 0.1*B/T + 0.016*(B/T)^2;
SA = 2*pi/4*T*L; %projected area of pontoon for two pontoons

%% Linear Drag Terms
%Total Speed
U = sqrt(u^2+v^2);

Xu = 0;
Yv = -0.5*rho*abs(v)*2*Cdc*SA; %20 was the last working number %from SNAME 1950, x2 for two cylinders
%Nr = -0.5*pi*rho*U*T^2*L^2;
Nr = -pi*rho*U*T^2*L^2*.065;
Nv = -pi*rho*U*T^2*L*.01;
Yr = pi*rho*U*T^2*L*0.2;  %from Newman approximation in Lewandowski

%% Nonlinear Drag Terms

% Drag and Moment due to drag on entire vessel - includes nonlinear and
% linear drag terms
D_port = 0.5*(0.44*u_port^3 - 0.01*u_port^2 + 19*u_port);     % Can assume that this equation also takes into account Xu - so set Xu=0
D_stbd = 0.5*(0.44*u_stbd^3 - 0.01*u_stbd^2 + 19*u_stbd);     % Can assume that this equation also takes into account Xu - so set Xu=0

tau_drag = [-(D_port + D_stbd); 0; (D_stbd - D_port)*p_bar];

Xuu = 0;

%% Maneuvering Coefficient Matrices
% Added Mass Matrix
M = [(m - Xudot)      0              0;...
    0               (m - Yvdot)     (m*xg - Yrdot);...
    0               (m*xg - Nvdot)  (Iz - Nrdot)];

%Centripetal and Added Mass Centripetal force matrices
% C_RB = [
%     0                  0                0
%     0                  0                0
%     0                  0                0
%     ];

% C_RB = [
%     0                  0                -m*(xg*r + v)
%     0                  0                -m*(yg*r - u)
%     m*(xg*r + v)       m*(yg*r - u)     0
%     ];

% C_A = -[ %negative originally
%     0                               0           0
%     0                               0           0
%     0                               0           0
%     ];

% Negating centripetal acceleration for test
C_RB = 0;
C_A = 0;

D = -[Xu  0   0;...
      0   Yv  Yr;...
      0   Nv  Nr];

% Nonlinear Drag Coefficients
D_N = -[Xuu*u   0                       0;...
        0       0                       0;...
        0       0                       0];
    
%% Calculate the port and starboard force vectors
tau_port = -(C_RB + C_A + D + D_N)*state_port;
tau_stbd = -(C_RB + C_A + D + D_N)*state_stbd;


%% Sum the force vectors
tau_tot = tau + tau_drag + tau_port + tau_stbd...
    + cross(r_port,[tau_port(1);tau_port(2);0]) + ...
    cross(r_stbd,[tau_stbd(1);tau_stbd(2);0]);

% Calculate the time derivative of the state vector

accel = M\tau_tot;

%% Separate output

surgeAccel = accel(1);
swayAccel = accel(2);
yawAccel = accel(3);

end

== matlab function RobotX_SLAMonly/Main FSM/SLAM/Models for prediction/Model14/Port Thruster Model ==
  data: portMP input; F_surge output; portAzimuth input; F_sway output; Torque output
function [F_surge,F_sway,Torque]  = PortThruster(portMP,portAzimuth)
%Approximation for Starboard Force and Moment with the input motor power
%and azimuth angle of thruster

%Longitudinal distance from center of mass
longDist =1.007;           %m

%Axial distance from center of mass
axialDist=1.485;            %m

%% Piece-wise thrust calculation

if portMP <= -51.0119
    F = .9140*portMP + 40;
elseif portMP >= 26.8367
    F = 1.658*portMP - 41.01;
else
    F = .12987*portMP;
end

%% Force components
F_surge=F*cos(portAzimuth*pi/180);       %N
F_sway=F*sin(portAzimuth*pi/180);       %N

%% Torque calculation

Torque = F_surge*longDist - F_sway*axialDist;   %N.m

end

== matlab function RobotX_SLAMonly/Main FSM/SLAM/Models for prediction/Model14/Stbd Thruster Model ==
  data: stbdMP input; F_surge output; stbdAzimuth input; F_sway output; Torque output
function [F_surge,F_sway,Torque]  = StarBoardThruster(stbdMP,stbdAzimuth)
%Approximation for Starboard Force and Moment with the input motor power
%and azimuth angle of thruster

%Longitudinal distance from center of mass
longDist =1.007;           %m

%Axial distance from center of mass
axialDist=1.485;            %m

%% Piece-wise thrust calculation

if stbdMP <= -51.0119
    F = .9140*stbdMP + 40;
elseif stbdMP >= 26.8367
    F = 1.658*stbdMP - 41.01;
else
    F = .12987*stbdMP;
end

%% Force components
F_surge=F*cos(stbdAzimuth*pi/180);       %N
F_sway=F*sin(stbdAzimuth*pi/180);       %N

%% Torque calculation

Torque = -F_surge*longDist - F_sway*axialDist;   %N.m

end
